simulink model "luoji1"  (Simulink 7.6)
settings: Solver=ode4  StartTime=0  StopTime=inf  FixedStep=0.001  RelTol=1e-3
settings Model: Creator=Administrator  LastModifiedBy=Administrator  SimulationMode=external  BufferReuse=off
settings OptimizationCC: BlockReduction=off  OptimizeBlockIOStorage=off  BufferReuse=off  ExpressionFolding=off  LocalBlockOutputs=off
settings HardwareCC: ProdIntDivRoundTo=Zero  ProdEndianess=LittleEndian  ProdHWDeviceType=Generic->32-bit x86 compatible
settings RTWCC: SystemTargetFile=xpctarget.tlc  TemplateMakefile=xpc_default_tmf  Description=xPC Target  ProcessScript=xpctarget_make_rtw_hook  RTWCompilerOptimization=On
settings xpcTargetCC: TargetFcnLib=ansi_tfl_table_tmw.mat  TargetFunctionLibrary=XPC_BLAS  ERTCodeCoverageTool=None  ParMdlRefBuildCompliant=on  CombineSignalStateStructs=off  PortableWordSizes=off  xPCLoadParamSetFile=off  xPCConcurrentTasks=off  xPCEnableSFAnimation=off

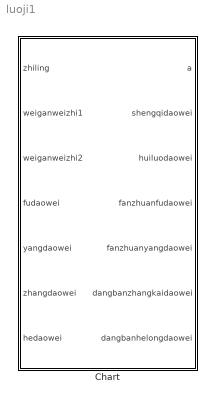
== system luoji1 ==
  Chart : Stateflow chart  TreatAsAtomicUnit=on

== stateflow chart Chart ==
  state start
    entry:
    a=0;
  state on1
    entry:
    a=1;
  state on2
    entry:
    a=2;
  state on3
    entry:
    a=3;
  state on4
    entry:
    a=4;
  state on5
    entry:
    a=5;
  state on6
    entry:
    a=6;
  state off1
    entry:
    a=0;
    shengqidaowei=1;
    huiluodaowei=0;
  state off2
    entry:
    a=0;
    shengqidaowei=0;
    huiluodaowei=1;
  state off3
    entry:
    a=0;
    fanzhuanfudaowei=1;
    fanzhuanyangdaowei=0;
  state off4
    entry:
    a=0;
    fanzhuanfudaowei=0;
    fanzhuanyangdaowei=1;
  state off5
    entry:
    a=0;
    dangbanzhangkaidaowei=1
    dangbanhelongdaowei=0;
  state off6
    entry:
    a=0;
    dangbanhelongdaowei=1;
    dangbanzhangkaidaowei=0;
  (default) -> start
  start -> (junction 16)
  (junction 16) -> on1 [order 1] : [zhiling==1]
  (junction 16) -> on2 [order 2] : [zhiling==2]
  (junction 16) -> on3 [order 3] : [zhiling==3]
  (junction 16) -> on4 [order 4] : [zhiling==4]
  (junction 16) -> on5 [order 5] : [zhiling==5]
  (junction 16) -> on6 [order 6] : [zhiling==6]
  on1 -> off1 : [weiganweizhi1==1]
  on2 -> off2 : [weiganweizhi2==2]
  on3 -> off3 : [fudaowei>=5200]
  on4 -> off4 : [yangdaowei<=1500]
  on5 -> off5 : [zhangdaowei>=4900]
  on6 -> off6 : [hedaowei<=1400]
  off1 -> start : after(2,tick)
  off2 -> start : after(2,tick)
  off3 -> start : after(2,tick)
  off4 -> start : after(2,tick)
  off5 -> start : after(2,tick)
  off6 -> start : after(2,tick)
  data: a output double; zhiling input double; weiganweizhi1 input double; weiganweizhi2 input double; fudaowei input double; yangdaowei input double; zhangdaowei input double; hedaowei input double; shengqidaowei output double; huiluodaowei output double; fanzhuanfudaowei output double; fanzhuanyangdaowei output double; dangbanzhangkaidaowei output double; dangbanhelongdaowei output double
